simulink library "allocator_lib"  (R2018b)
settings: Solver=VariableStepAuto  StartTime=0.0  StopTime=10.0  RelTol=1e-3
undefined symbols (not defined in the file or in its folder): fswParams
libraries: rwa_allocation_lib x1, torque_2_rpm_lib x1
settings Model: Creator=taylorreynolds  LastModifiedBy=taylorreynolds

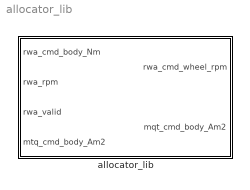
== system allocator_lib ==
  allocator_lib : Subsystem

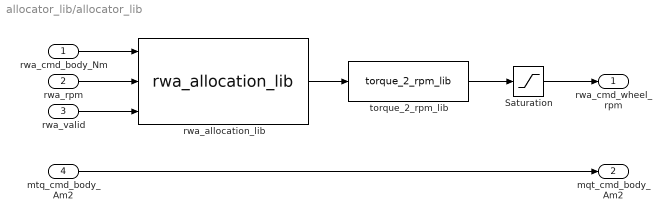
== system allocator_lib/allocator_lib ==
  rwa_cmd_body_Nm : Inport
  rwa_rpm : Inport  Port=2
  rwa_valid : Inport  Port=3
  mtq_cmd_body_Am2 : Inport  Port=4
  Saturation : Saturate  UpperLimit=fswParams.actuators.rwa.max_RPM  LowerLimit=-fswParams.actuators.rwa.max_RPM
  rwa_allocation_lib : rwa_allocation_lib/rwa_allocation_lib  SystemSampleTime=-1
  torque_2_rpm_lib : torque_2_rpm_lib/torque_2_rpm_lib  SystemSampleTime=-1
  rwa_cmd_wheel_rpm : Outport
  mqt_cmd_body_Am2 : Outport  Port=2
  wires:
  rwa_cmd_body_Nm/1 -> rwa_allocation_lib/1
  rwa_allocation_lib/1 -> torque_2_rpm_lib/1
  torque_2_rpm_lib/1 -> Saturation/1
  rwa_rpm/1 -> rwa_allocation_lib/2
  rwa_valid/1 -> rwa_allocation_lib/3
  mtq_cmd_body_Am2/1 -> mqt_cmd_body_Am2/1
  Saturation/1 -> rwa_cmd_wheel_rpm/1
